simulink library "RisingEdgeTimer"  (R2020b)
settings: Solver=VariableStepAuto  StartTime=0.0  StopTime=10.0  RelTol=1e-3
settings Model: Creator=GW00166368  LastModifiedBy=GW00166368

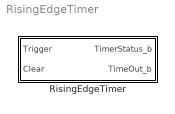
== system RisingEdgeTimer ==
  RisingEdgeTimer : Subsystem  mask(RisingEdgeTimer){MaxCnt=0}
      mask help: 若MaxCycles~=0，当Trigger（Boolean）端口检测到上升沿后，开始计数，输出TimerStatus_b（Boolean）为true。当计数达到MaxCnt时，或Clear（Boolean）端口检测到true后，计数器清零，TimerStatus_b输出false。若MaxCycles==0，则只能由Clear端口输入true将输出置false。当因为计数达到MaxCnt而导致TimerStatus_b输出false时，且Trigger端口输入在此期间始终为true，则TimeOut_b端口置true，直到Trigger端口输入false，或者clear端口输入true。
      mask Help:
      | 典型用法1
      | 功能抑制计时器，当检测到某条件达成后，抑制某功能一段时间。

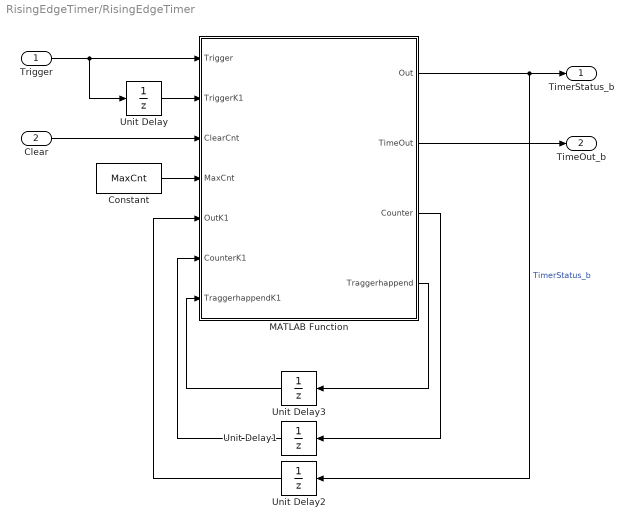
== system RisingEdgeTimer/RisingEdgeTimer ==
  Trigger : Inport  OutDataTypeStr=boolean
  Clear : Inport  Port=2  OutDataTypeStr=boolean
  Constant : Constant  Value=MaxCnt  OutDataTypeStr=uint16
  MATLAB Function : MATLAB Function  TreatAsAtomicUnit=on
  Unit Delay{,1..3} (4 alike) : UnitDelay  SampleTime=-1  HasFrameUpgradeWarning=on
  TimerStatus_b : Outport  OutDataTypeStr=boolean
  TimeOut_b : Outport  Port=2  OutDataTypeStr=boolean
  wires:
  Unit Delay2/1 -> MATLAB Function/5(OutK1)
  MATLAB Function/1(Out) -> Unit Delay2/1, TimerStatus_b/1  "TimerStatus_b"
  Constant/1 -> MATLAB Function/4(MaxCnt)
  MATLAB Function/3(Counter) -> Unit Delay1/1
  Unit Delay/1 -> MATLAB Function/2(TriggerK1)
  Unit Delay1/1 -> MATLAB Function/6(CounterK1)
  Trigger/1 -> MATLAB Function/1(Trigger), Unit Delay/1
  Clear/1 -> MATLAB Function/3(ClearCnt)
  MATLAB Function/2(TimeOut) -> TimeOut_b/1
  MATLAB Function/4(Traggerhappend) -> Unit Delay3/1
  Unit Delay3/1 -> MATLAB Function/7(TraggerhappendK1)

== matlab function RisingEdgeTimer/MATLAB Function ==
  data: Trigger input boolean; Out output boolean; TimeOut output boolean; TriggerK1 input boolean; ClearCnt input boolean; MaxCnt input uint16; OutK1 input boolean; CounterK1 input uint16; Counter output uint16; TraggerhappendK1 input boolean; Traggerhappend output boolean
function [Out,TimeOut,Counter,Traggerhappend] = RisingEdgeTimer(Trigger,TriggerK1, ClearCnt, MaxCnt,OutK1, CounterK1,TraggerhappendK1)
%#codegen
TimeOut=false;
Traggerhappend=TraggerhappendK1;
if MaxCnt~=0
    if (Trigger==1)&&(TriggerK1==0)
        Counter = MaxCnt;
        Traggerhappend=true;
    elseif CounterK1 > 0x0
        Counter = CounterK1 - uint16(1);
    else
        Counter = CounterK1;
    end 
    if ClearCnt
        Traggerhappend=false;
        Counter = uint16(0);
    end
    if Counter > 0x0
        Out = true;
    else
        Out = false;
    end
else
    Counter = uint16(0);
    if (Trigger==1)&&(TriggerK1==0)
        Out=true;
    else
        Out=OutK1;
    end
    if ClearCnt
        Out=false;
    end
end
if Counter==uint16(0) && Trigger==1 && Traggerhappend
    TimeOut=true;
end 
if Trigger==0
    Traggerhappend=false;
end
end
